simulink model "ACSI_Aero_Simulink_SS_1"  (R2018a)
settings: Solver=ode1  StartTime=0.0  StopTime=inf  FixedStep=0.002  RelTol=1e-3  EnableMultiTasking=on
PreLoadFcn:
  | quanser_aero_state_space
values from neighbouring files (symbols this model uses):
  A = [0 0 1 0 ... (first row only)    [Lab1_dynDecPID.m]    (also in quanser_aero_state_space.m)
  B = [0 0 ... (first row only)    [Lab1_dynDecPID.m]    (also in quanser_aero_state_space.m)
  C = eye(2,4)    [Lab1_dynDecPID.m]    (also in quanser_aero_state_space.m)
  K = lqr(A, B, Q, R)    [quanser_aero_state_space.m]
  L = place(A', C', po)'    [quanser_aero_state_space.m]
undefined symbols (not defined in the file or in its folder): HIL, qc_get_step_size
libraries: quarc_library x8
settings Model: SimulationMode=external  ExtModeTrigDuration=200000  Creator=MLevis  LastModifiedBy=Joe
settings SolverCC: PositivePriorityOrder=on
settings DataIOCC: LimitDataPoints=on  SaveFormat=Array
settings OptimizationCC: LifeSpan=inf
settings DebuggingCC: SolverPrmCheckMsg=warning  SFUnexpectedBacktrackingDiag=warning  SFNoUnconditionalDefaultTransitionDiag=warning  SFExecutionAtInitializationDiag=none
settings HardwareCC: ProdBitPerPointer=32  ProdBitPerSizeT=32  ProdBitPerPtrDiffT=32  ProdLargestAtomicFloat=None  ProdIntDivRoundTo=Undefined  ProdEndianess=Unspecified  ProdWordSize=32  ProdHWDeviceType=32-bit Generic
settings ModelReferenceCC: PropagateSignalLabelsOutOfModel=off
settings RTWCC: SystemTargetFile=quarc_win64.tlc  TemplateMakefile=quarc_default_tmf  Description=QUARC Win64 Target
settings CodeAppCC: StateflowObjectComments=on
settings STFCustomTargetCC: TargetPreCompLibLocation=C:\PROGRA~3\QUARC\lib\2018a\win64\release  ConcurrentExecutionCompliant=on  GeneratePreprocessorConditionals=Disable all  SystemTargetFile=quarc_win64.tlc
settings GRTTargetCC: TargetPreCompLibLocation=C:\PROGRA~3\QUARC\lib\2018a\win64\release  TargetLangStandard=C89/C90 (ANSI)  ParMdlRefBuildCompliant=off  CompOptLevelCompliant=off  GeneratePreprocessorConditionals=Disable all  CombineOutputUpdateFcns=off  MatFileLogging=off  CPPClassGenCompliant=off  GRTInterface=on  UseToolchainInfoCompliant=off  ExtMode=on  ExtModeMexFile=quarc_comm
settings ConfigComp: CovMetricSettings=dw  CovHtmlReporting=on  CovSaveCumulativeToWorkspaceVar=on  CovSaveSingleToWorkspaceVar=on  CovExternalEMLEnable=off  CovSFcnEnable=off

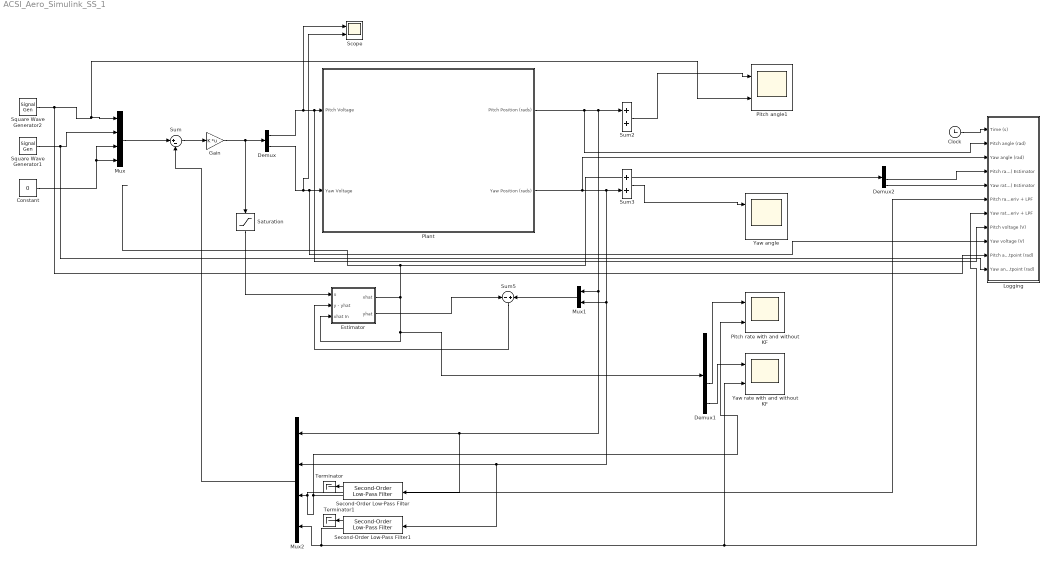
== system ACSI_Aero_Simulink_SS_1 ==
  Clock : Clock
  Constant : Constant  Value=0
  Demux : Demux  Outputs=2
  Demux1 : Demux
  Demux2 : Demux
  "Estimator " : Subsystem
  Gain : Gain  Gain=K  Multiplication=Matrix(K*u) (u vector)
  Logging : Subsystem
  Mux : Mux
  Mux1 : Mux  Inputs=2
  Mux2 : Mux
  Pitch angle1 : Scope  NumInputPorts=2
  Pitch rate with and without KF : Scope  NumInputPorts=2
  Plant : Subsystem
  Saturation : Saturate  UpperLimit=24  LowerLimit=-24
  Scope : Scope  NumInputPorts=2
  Second-Order Low-Pass Filter : quarc_library/Continuous/Second-Order Low-Pass Filter  params_source=Internal (dialog parameters)  input_width=50  input_zeta=.8  input_init=0
  Second-Order Low-Pass Filter1 : quarc_library/Continuous/Second-Order Low-Pass Filter  params_source=Internal (dialog parameters)  input_width=50  input_zeta=.8  input_init=0
  Square Wave Generator1 : SignalGenerator  WaveForm=square  Amplitude=pi/4  Frequency=.5  Units=rad/sec
  Square Wave Generator2 : SignalGenerator  WaveForm=square  Amplitude=pi/6  Frequency=.4  Units=rad/sec
  Sum : Sum  Inputs=|+-
  Sum2 : Sum
  Sum3 : Sum
  Sum5 : Sum  Inputs=-|+
  Terminator : Terminator
  Terminator1 : Terminator
  Yaw angle : Scope  NumInputPorts=2
  "Yaw rate with and without KF " : Scope  NumInputPorts=2
  wires:
  Sum3/1 -> Yaw angle/1
  Sum2/1 -> Pitch angle1/1
  Square Wave Generator2/1 -> Logging/10(Pitch angle setpoint (rad)), Mux/1, Pitch angle1/2
  Constant/1 -> Mux/4, Mux/3
  Mux/1 -> Sum/1
  Demux/1 -> Scope/1, Logging/8(Pitch voltage (V)), Plant/1(Pitch Voltage)
  Demux/2 -> Scope/2, Logging/9(Yaw voltage (V)), Plant/2(Yaw Voltage)
  Sum/1 -> Gain/1
  Mux1/1 -> Sum5/2
  Plant/2(Yaw Position (rads)) -> Logging/3("Yaw angle (rad) "), Second-Order Low-Pass Filter1/1, Mux2/2, Mux1/2, Sum3/2
  Plant/1(Pitch Position (rads)) -> Logging/2(Pitch angle (rad)), Second-Order Low-Pass Filter/1, Mux2/1, Mux1/1, Sum2/1
  Second-Order Low-Pass Filter/2 -> Logging/6(Pitch rate (rad/s) Deriv + LPF), Mux2/3, Pitch rate with and without KF/2
  Second-Order Low-Pass Filter1/2 -> Logging/7(Yaw rate (rad/s) Deriv + LPF), "Yaw rate with and without KF "/2, Mux2/4
  Demux1/4 -> "Yaw rate with and without KF "/1
  Second-Order Low-Pass Filter/1 -> Terminator/1
  Second-Order Low-Pass Filter1/1 -> Terminator1/1
  Mux2/1 -> Sum/2
  Demux1/3 -> Pitch rate with and without KF/1
  Square Wave Generator1/1 -> Logging/11(Yaw angle setpoint (rad)), Mux/2
  Clock/1 -> Logging/1("Time (s) ")
  Demux2/3 -> Logging/4(Pitch rate (rad/s) Estimator)
  Demux2/4 -> Logging/5(Yaw rate (rad/s) Estimator)
  Gain/1 -> Saturation/1, Demux/1
  "Estimator "/1(xhat) -> Demux2/1, "Estimator "/3(xhat In), Demux1/1
  Saturation/1 -> "Estimator "/1(u)
  Sum5/1 -> "Estimator "/2(y - yhat)
  "Estimator "/2(yhat) -> Sum5/1

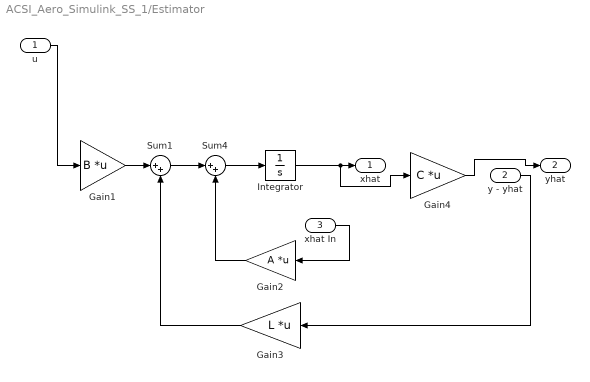
== system ACSI_Aero_Simulink_SS_1/Estimator  ==
  u : Inport
  y - yhat : Inport  Port=2
  xhat In : Inport  Port=3
  Gain1 : Gain  Gain=B  Multiplication=Matrix(K*u) (u vector)
  Gain2 : Gain  Gain=A  Multiplication=Matrix(K*u) (u vector)
  Gain3 : Gain  Gain=L  Multiplication=Matrix(K*u) (u vector)
  Gain4 : Gain  Gain=C  Multiplication=Matrix(K*u) (u vector)
  Integrator : Integrator
  Sum1 : Sum  Inputs=|++
  Sum4 : Sum  Inputs=|++
  xhat : Outport
  yhat : Outport  Port=2
  wires:
  Integrator/1 -> Gain4/1, xhat/1
  Sum4/1 -> Integrator/1
  Gain1/1 -> Sum1/1
  xhat In/1 -> Gain2/1
  Sum1/1 -> Sum4/1
  Gain3/1 -> Sum1/2
  Gain4/1 -> yhat/1
  Gain2/1 -> Sum4/2
  y - yhat/1 -> Gain3/1
  u/1 -> Gain1/1

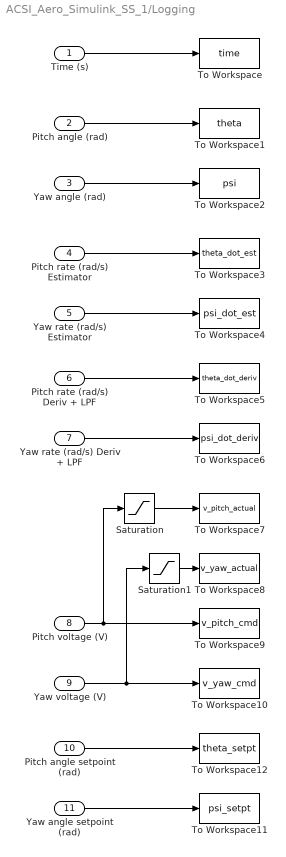
== system ACSI_Aero_Simulink_SS_1/Logging ==
  "Time (s) " : Inport
  Pitch angle (rad) : Inport  Port=2
  "Yaw angle (rad) " : Inport  Port=3
  Pitch rate (rad/s) Estimator : Inport  Port=4
  Yaw rate (rad/s) Estimator : Inport  Port=5
  Pitch rate (rad/s) Deriv + LPF : Inport  Port=6
  Yaw rate (rad/s) Deriv + LPF : Inport  Port=7
  Pitch voltage (V) : Inport  Port=8
  Yaw voltage (V) : Inport  Port=9
  Pitch angle setpoint (rad) : Inport  Port=10
  Yaw angle setpoint (rad) : Inport  Port=11
  Saturation : Saturate  UpperLimit=24  LowerLimit=-24
  Saturation1 : Saturate  UpperLimit=24  LowerLimit=-24
  To Workspace : ToWorkspace  VariableName=time  SampleTime=-1
  To Workspace1 : ToWorkspace  VariableName=theta  SampleTime=-1
  To Workspace10 : ToWorkspace  VariableName=v_yaw_cmd  SampleTime=-1
  To Workspace11 : ToWorkspace  VariableName=psi_setpt  SampleTime=-1
  To Workspace12 : ToWorkspace  VariableName=theta_setpt  SampleTime=-1
  To Workspace2 : ToWorkspace  VariableName=psi  SampleTime=-1
  To Workspace3 : ToWorkspace  VariableName=theta_dot_est  SampleTime=-1
  To Workspace4 : ToWorkspace  VariableName=psi_dot_est  SampleTime=-1
  To Workspace5 : ToWorkspace  VariableName=theta_dot_deriv  SampleTime=-1
  To Workspace6 : ToWorkspace  VariableName=psi_dot_deriv  SampleTime=-1
  To Workspace7 : ToWorkspace  VariableName=v_pitch_actual  SampleTime=-1
  To Workspace8 : ToWorkspace  VariableName=v_yaw_actual  SampleTime=-1
  To Workspace9 : ToWorkspace  VariableName=v_pitch_cmd  SampleTime=-1
  wires:
  "Time (s) "/1 -> To Workspace/1
  Pitch angle (rad)/1 -> To Workspace1/1
  "Yaw angle (rad) "/1 -> To Workspace2/1
  Pitch rate (rad/s) Estimator/1 -> To Workspace3/1
  Yaw rate (rad/s) Estimator/1 -> To Workspace4/1
  Pitch rate (rad/s) Deriv + LPF/1 -> To Workspace5/1
  Yaw rate (rad/s) Deriv + LPF/1 -> To Workspace6/1
  Yaw voltage (V)/1 -> Saturation1/1, To Workspace10/1
  Pitch voltage (V)/1 -> Saturation/1, To Workspace9/1
  Saturation/1 -> To Workspace7/1
  Saturation1/1 -> To Workspace8/1
  Pitch angle setpoint (rad)/1 -> To Workspace12/1
  Yaw angle setpoint (rad)/1 -> To Workspace11/1

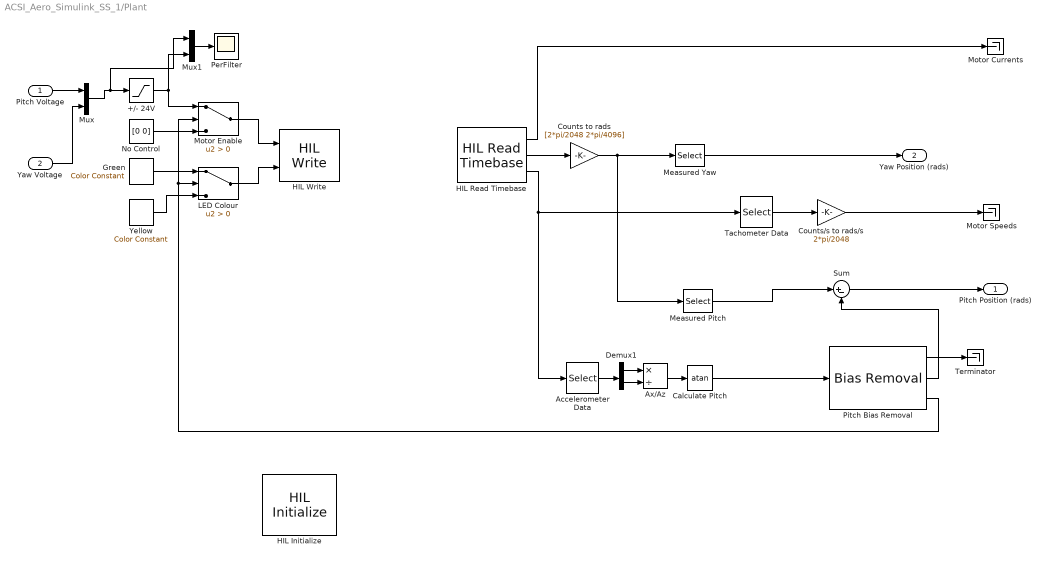
== system ACSI_Aero_Simulink_SS_1/Plant ==
  Pitch Voltage : Inport
  Yaw Voltage : Inport  Port=2
  +/- 24V : Saturate  UpperLimit=24  LowerLimit=-24
  Accelerometer Data : Selector  InputPortWidth=4  IndexOptions=Index vector (dialog)  Indices=[1 2]  OutputSizes=1
  Ax/Az : Product  Inputs=*/
  Calculate Pitch : Trigonometry  Operator=atan
  Counts to rads : Gain  Gain=[2*pi/2048 2*pi/4096]
  Counts/s to rads/s : Gain  Gain=2*pi/2048
  Demux1 : Demux  Outputs=2
  Green : quarc_library/Sources/Signals/Color Constant  color=[0 1 0]
      settings: SourceProductName=QUARC Targets
  HIL Initialize : quarc_library/Data Acquisition/Generic/Configuration/HIL Initialize  Priority=-99  object_name=HIL-1  board_type=quanser_aero_usb  board_number=0  board_options=""  exclusive=off  active=off  hardware_clocks=[0]  clock_modes=[]  initial_clock_frequencies=[]  set_clock_params_at_start=off  set_clock_params_at_switch_in=off  set_clock_frequencies_at_start=off  set_clock_frequencies_at_switch_in=off  analog_input_channels=[0:1]  analog_input_configurations=0  analog_input_maximums=3  analog_input_minimums=-3  set_analog_input_params_at_start=off  set_analog_input_params_at_switch_in=off  analog_output_channels=[0:1]  analog_output_maximums=24  analog_output_minimums=-24  initial_analog_outputs=[0]  final_analog_outputs=[0]  watchdog_analog_outputs=[0]  set_analog_output_params_at_start=off  set_analog_output_params_at_switch_in=off  set_analog_outputs_at_start=on  set_analog_outputs_at_switch_in=off  set_analog_outputs_at_terminate=on  set_analog_outputs_at_switch_out=off  set_analog_outputs_on_watchdog=on  digital_input_channels=[]  digital_output_channels=[0:1]  digital_output_configuration=[]  initial_digital_outputs=[1]  final_digital_outputs=[0]  watchdog_digital_outputs=[0]  set_digital_output_params_at_start=off  set_digital_output_params_at_switch_in=off  set_digital_outputs_at_start=on  set_digital_outputs_at_switch_in=off  set_digital_outputs_at_terminate=on  set_digital_outputs_at_switch_out=off  set_digital_outputs_on_watchdog=on  encoder_channels=[0:3]  quadrature=[4]  encoder_filter_frequency=[]  initial_encoder_counts=[0]  set_encoder_params_at_start=off  set_encoder_params_at_switch_in=off  set_encoder_counts_at_start=on  set_encoder_counts_at_switch_in=off  pwm_channels=[]  pwm_modes=[]  pwm_frequency=[]  pwm_configuration=[]  pwm_alignment=[]  pwm_polarity=[]  pwm_leading_deadband=[]  pwm_trailing_deadband=[]  initial_pwm_outputs=[]  final_pwm_outputs=[]  watchdog_pwm_outputs=[]  set_pwm_params_at_start=off  set_pwm_params_at_switch_in=off  set_pwm_outputs_at_start=off  set_pwm_outputs_at_switch_in=off  set_pwm_outputs_at_terminate=off  set_pwm_outputs_at_switch_out=off  set_pwm_outputs_on_watchdog=off  other_output_channels=[11000:11002]  initial_other_outputs=[0 1 0]  final_other_outputs=[1 0 0]  watchdog_other_outputs=[0 0 1]  set_other_outputs_at_start=on  set_other_outputs_at_switch_in=off  set_other_outputs_at_terminate=on  set_other_outputs_at_switch_out=off  set_other_outputs_on_watchdog=on
  HIL Read Timebase : quarc_library/Data Acquisition/Generic/Timebases/HIL Read Timebase  object_name=HIL-1  clock=0  analog_channels=[0:1]  encoder_channels=[2:3]  digital_channels=[]  other_channels=[4000 4002 14000 14001]  samples_in_buffer=max(ceil(1/qc_get_step_size), 1)  active=on  vector_output=on  data_type_mode=Inherit via back propagation  encoder_data_type=double  digital_data_type=boolean
  HIL Write : quarc_library/Data Acquisition/Generic/Immediate I//O/HIL Write  object_name=HIL-1  analog_channels=[0:1]  pwm_channels=[]  digital_channels=[]  other_channels=[11000:11002]  sample_time=-1  active=off  vector_input=on
  LED Colour : Switch  Criteria=u2 > Threshold
  Measured Pitch : Selector  InputPortWidth=2  IndexOptions=Index vector (dialog)  Indices=[1]  OutputSizes=1
  Measured Yaw : Selector  InputPortWidth=2  IndexOptions=Index vector (dialog)  Indices=[2]  OutputSizes=1
  Motor Currents : Terminator
  Motor Enable : Switch  Criteria=u2 > Threshold
  Motor Speeds : Terminator
  Mux : Mux  Inputs=2
  Mux1 : Mux  Inputs=2
  No Control : Constant  Value=[0 0]
  PerFilter : Scope
  Pitch Bias Removal : quarc_library/Discrete/Bias Removal  start_time=0  end_time=1  switch_id=0  sample_time=qc_get_step_size
      settings: SourceProductName=QUARC Targets
  Sum : Sum  Inputs=|+-
  Tachometer Data : Selector  InputPortWidth=4  IndexOptions=Index vector (dialog)  Indices=[3 4]  OutputSizes=1
  Terminator : Terminator
  Yellow : quarc_library/Sources/Signals/Color Constant  color=[1 1 0]
      settings: SourceProductName=QUARC Targets
  Pitch Position (rads) : Outport
  Yaw Position (rads) : Outport  Port=2
  wires:
  Pitch Bias Removal/3 -> Motor Enable/2, LED Colour/2
  +/- 24V/1 -> Mux1/2, Motor Enable/1
  Motor Enable/1 -> HIL Write/1
  Green/1 -> LED Colour/1
  Yellow/1 -> LED Colour/3
  LED Colour/1 -> HIL Write/2
  No Control/1 -> Motor Enable/3
  Tachometer Data/1 -> Counts/s to rads/s/1
  Demux1/1 -> Ax/Az/1
  Demux1/2 -> Ax/Az/2
  HIL Read Timebase/2 -> Counts to rads/1
  Calculate Pitch/1 -> Pitch Bias Removal/1
  Counts/s to rads/s/1 -> Motor Speeds/1
  HIL Read Timebase/1 -> Motor Currents/1
  Accelerometer Data/1 -> Demux1/1
  HIL Read Timebase/3 -> Accelerometer Data/1, Tachometer Data/1
  Counts to rads/1 -> Measured Pitch/1, Measured Yaw/1
  Ax/Az/1 -> Calculate Pitch/1
  Pitch Bias Removal/2 -> Sum/2
  Pitch Voltage/1 -> Mux/1
  Yaw Voltage/1 -> Mux/2
  Mux/1 -> Mux1/1, +/- 24V/1
  Pitch Bias Removal/1 -> Terminator/1
  Sum/1 -> Pitch Position (rads)/1
  Measured Pitch/1 -> Sum/1
  Measured Yaw/1 -> Yaw Position (rads)/1
  Mux1/1 -> PerFilter/1
